simulink model "Helicopter_sol"  (R2023b)
settings: Solver=ode3  StartTime=0.0  StopTime=20  FixedStep=0.01  RelTol=1e-3
values from neighbouring files (symbols this model uses):
  A = [ -0.4 ,   0 , -0.01 ... (first row only)    [Helicopter_DT_par_sol.m]    (also in Helicopter_par_sol.m)
  B = [ 6.3 ; 0 ; 9.8 ]    [Helicopter_DT_par_sol.m]    (also in Helicopter_par_sol.m)
  C = [ 0 , 0 , 1 ]    [Helicopter_DT_par_sol.m]    (also in Helicopter_par_sol.m)
  K = lqi(sys_DT,Q,R)    [Helicopter_DT_par_sol.m]    (also in Helicopter_par_sol.m = lqr(A,B,Q,R))
  K_E = lqi(sysCT,Q_E,R)    [Helicopter_par_sol.m]
libraries: simulink_extras x2
settings Model: Creator=jerome  LastModifiedBy=jerome
settings ModelReferenceCC: EnableRefExpFcnMdlSchedulingChecks=on

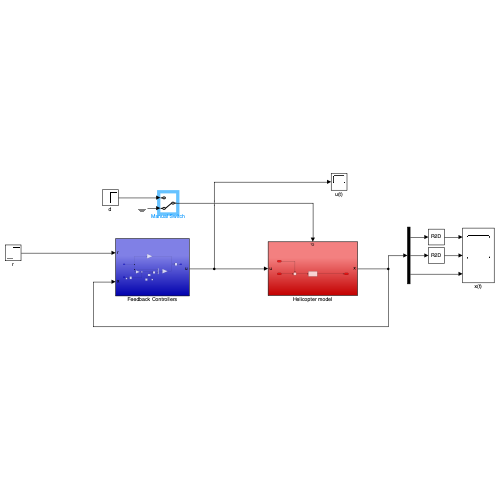
[thumbnail: Simulink's stored preview of the top-level diagram]
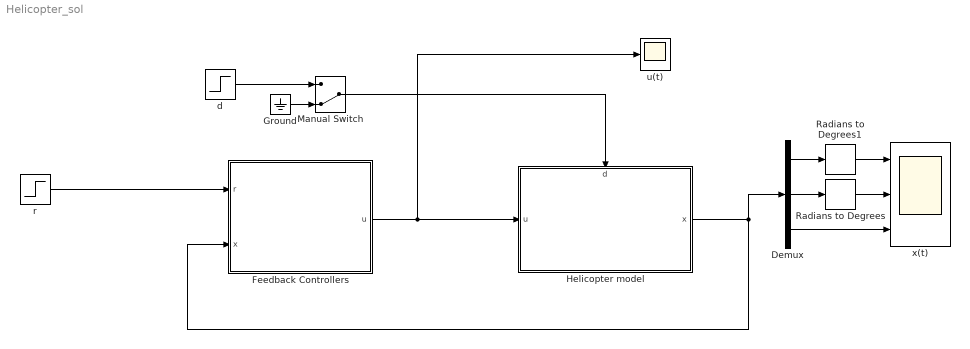
== system Helicopter_sol ==
  Demux : Demux  Outputs=3
  Feedback Controllers : Subsystem
  Ground : Ground
  Helicopter model : Subsystem
      settings: PortSchema="{\"entries\":[{\"content\":{\"sides\":[{\"content\":{\"connectorIds\":[\"In1\"]},\"type\":\"ConnectorPlacement.EquallySpacedRectSide\",\"uuid\":\"2518be5c-e170-4c0f-887d-4f71d374b130\"},{\"content\":{\"connectorIds\":[\"Out1\"],\"side\":\"RIGHT\"},\"type\":\"ConnectorPlacement.EquallySpacedRectSide\",\"uuid\":\"95cc49d7-73c3-454f-9e39-99756c6ced38\"},{\"content\":{\"connectorIds\":[\"In2\"],\"side\":\"TOP\"},\"type\":\"ConnectorPlacement.EquallySpacedRectSide\",\"uuid\":\"2ea20af2-734c-497d-bdc0-a9a861fe472b\"}]},\"type\":\"ConnectorPlacement.EquallySpacedConnector\",\"uuid\":\"0b247156-ce1f-410d-824c-75b8113742dd\"}],\"packageUris\":[\"http://schema.mathworks.com/mf0/Connector/R2020b\"],\"version\":\"1.0\"}"
  Manual Switch : ManualSwitch  CurrentSetting=0
  Radians to Degrees : simulink_extras/Transformations/Radians to Degrees
  Radians to Degrees1 : simulink_extras/Transformations/Radians to Degrees
  d : Step  Time=4  SampleTime=0
  r : Step  Time=8  After=10  SampleTime=0
  u(t) : Scope
  x(t) : Scope  NumInputPorts=3
  wires:
  Helicopter model/1(x) -> Demux/1, Feedback Controllers/2(x)
  Demux/2 -> Radians to Degrees/1
  Radians to Degrees/1 -> x(t)/2
  Radians to Degrees1/1 -> x(t)/1
  Feedback Controllers/1(u) -> u(t)/1, Helicopter model/1(u)
  Demux/3 -> x(t)/3
  Demux/1 -> Radians to Degrees1/1
  Manual Switch/1 -> Helicopter model/2(d)
  Ground/1 -> Manual Switch/2
  d/1 -> Manual Switch/1
  r/1 -> Feedback Controllers/1(r)

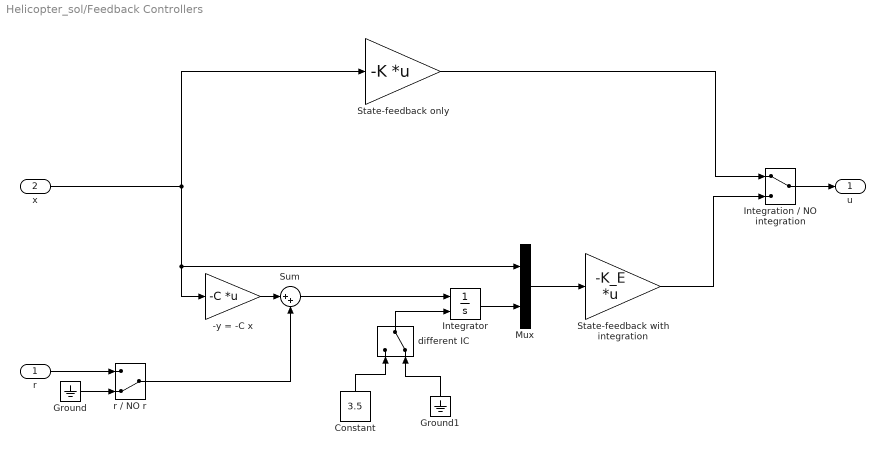
== system Helicopter_sol/Feedback Controllers ==
  r : Inport
  x : Inport  Port=2
  -y = -C x : Gain  Gain=-C  Multiplication=Matrix(K*u) (u vector)
  Constant : Constant  Value=3.5
  Ground : Ground
  Ground1 : Ground
  Integration / NO integration : ManualSwitch
  Integrator : Integrator  InitialConditionSource=external
  Mux : Mux  Inputs=2
  State-feedback only : Gain  Gain=-K  Multiplication=Matrix(K*u) (u vector)
  State-feedback with integration : Gain  Gain=-K_E  Multiplication=Matrix(K*u) (u vector)
  Sum : Sum  Inputs=|++
  different IC : ManualSwitch  CurrentSetting=0
  r / NO r : ManualSwitch  CurrentSetting=0
  u : Outport
  wires:
  x/1 -> -y = -C x/1, Mux/1, State-feedback only/1
  Integration / NO integration/1 -> u/1
  State-feedback only/1 -> Integration / NO integration/1
  State-feedback with integration/1 -> Integration / NO integration/2
  Mux/1 -> State-feedback with integration/1
  Integrator/1 -> Mux/2
  r/1 -> r / NO r/1
  Ground/1 -> r / NO r/2
  -y = -C x/1 -> Sum/1
  Sum/1 -> Integrator/1
  r / NO r/1 -> Sum/2
  different IC/1 -> Integrator/2
  Constant/1 -> different IC/1
  Ground1/1 -> different IC/2

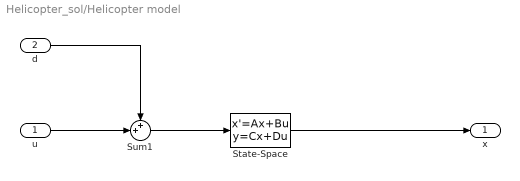
== system Helicopter_sol/Helicopter model ==
  u : Inport
  d : Inport  Port=2
  State-Space : StateSpace  A=A  B=B  C=eye(3)  D=zeros(3,1)  InitialCondition=[0;0;1]
  Sum1 : Sum  Inputs=++|
  x : Outport
  wires:
  State-Space/1 -> x/1
  Sum1/1 -> State-Space/1
  u/1 -> Sum1/2
  d/1 -> Sum1/1
